simulink model "gm_Model"  (R2025a)
settings: Solver=FixedStepDiscrete  StartTime=0.0  StopTime=80000/fs_in  RelTol=1e-3
undefined symbols (not defined in the file or in its folder): a, b, b_fixp, beta_retanh, c, cos_omega, cos_omega_fixp, diag_count, exp_omega, exp_omega_fixp, fixp_chebacc_frac, fixp_chebacc_ws, fixp_dsp_ws, fixp_eig_frac, fixp_eig_ws, fs_in, group_size, hann_table_fixp, image_seed, image_seed_fixp, J_ROM, k, K_ROM, lap_diags, lap_main, lap_main_fi, lap_offsets, lap_offsets_fi, lap_rest, lap_rest_fi, laplacian_diags_main, laplacian_diags_offsets, laplacian_diags_rest, lut_norm_x, lut_norm_y, magnitude, n_ch, n_layer, n_px, n_px_fi, nf, norm_gain_floor, power_iters, power_norm_scaling_factor_fixp, tau, tau_fixp, theta, theta_fixp
libraries: simulink x59, hdlsllib x36, hdlstreaminglib x4, hdlmdlgenlib x1, matrix_library x1, dspvision x1
(part 4 of 8)

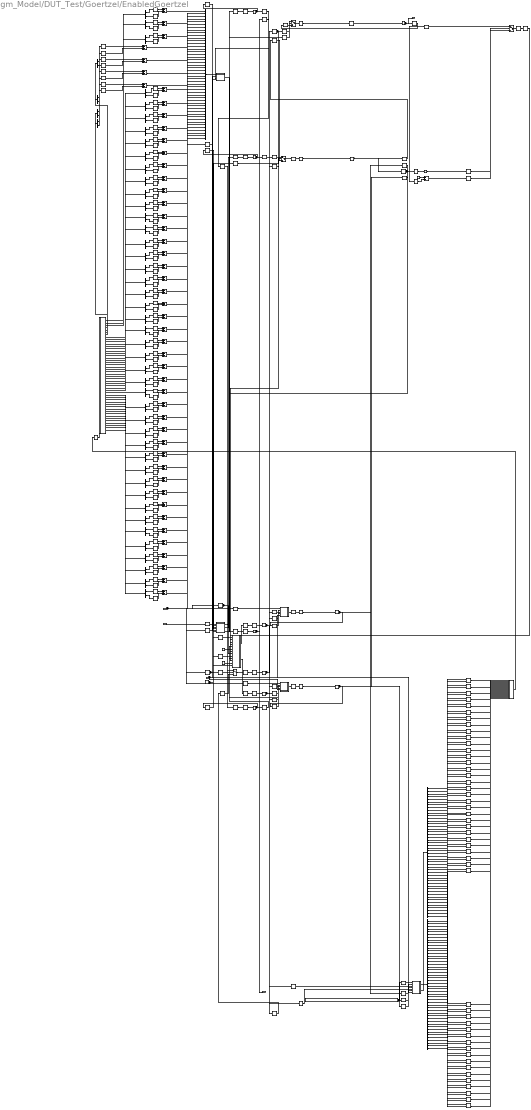
== system gm_Model/DUT_Test/Goertzel/EnabledGoertzel ==
  note: For Each
  note: For Each
  note: Symmetric Hann
  samples_in : Inport  OutDataTypeStr=fixdt(1, 12, 11)  PortDimensions=[1 48]  SampleTime=6.25e-05
  valid_in : Inport  Port=2  OutDataTypeStr=boolean  SampleTime=6.25e-05
  sch_ctr_199 : Inport  Port=3  OutDataTypeStr=uint8  SampleTime=3.125e-07
  Compare To Constant : simulink/Logic and Bit Operations/Compare To Constant  relop=<  const="fi(0,0,8,0,\"hex\",\"64\")"  OutDataTypeStr=boolean
  Constant : Constant  Value=[1.580322265625;1.6180419921875]  OutDataTypeStr=fixdt(1, 18, 13)  SampleTime=3.125e-07
  Constant1 : Constant  Value=0  OutDataTypeStr=fixdt(1, 18, 13)  SampleTime=3.125e-07
  Constant11 : Constant  Value=0  OutDataTypeStr=fixdt(1, 18, 13)  SampleTime=3.125e-07
  Constant12 : Constant  Value="complex(fi(\"numerictype\",numerictype(1,18,13),\"fimath\",fimath(\"RoundingMethod\", \"Nearest\",\"OverflowAction\", \"Saturate\",\"ProductMode\",\"FullPrecision\",\"SumMode\",\"FullPrecision\"),\"Value\",\"[0.7901611328125+0.6129150390625i;0.8089599609375+0.5877685546875i]\"))"  OutDataTypeStr=fixdt(1, 18, 13)  SampleTime=3.125e-07
  Constant2 : Constant  Value=199  OutDataTypeStr=uint8  SampleTime=3.125e-07
  Delay{,1..5,11..12,31,41} (10 alike) : RateTransition  InitialCondition=double(0)  OutPortSampleTimeOpt=Multiple of input port sample time  OutPortSampleTimeMultiple=200
  Delay1_absorbed : Delay  DelayLength=0
  Delay1_absorbed1 : Delay  DelayLength=0
  Delay1_absorbed2 : Delay  DelayLength=0
  Delay2_absorbed : Delay  DelayLength=0
  Delay2_enbsw : Switch  Criteria=u2 ~= 0  Threshold=double(0)  OutDataTypeStr=uint8  SampleTime=3.125e-07  SaturateOnIntegerOverflow=off  InputSameDT=off
  Delay3_absorbed : Delay  DelayLength=0
  Delay4_absorbed : Delay  DelayLength=0
  Delay4_enbsw : Switch  Criteria=u2 ~= 0  Threshold=double(0)  OutDataTypeStr=boolean  SampleTime=3.125e-07  SaturateOnIntegerOverflow=off  InputSameDT=off
  Delay_absorbed{,1..3} (4 alike) : Delay  DelayLength=0
  Delay_enbsw : Switch  Criteria=u2 ~= 0  Threshold=double(0)  OutDataTypeStr=boolean  SampleTime=3.125e-07  SaturateOnIntegerOverflow=off  InputSameDT=off
  HDL Counter : RateTransition  InitialCondition=double(0)  OutPortSampleTimeOpt=Multiple of input port sample time  OutPortSampleTimeMultiple=200
  HDL Counter_absorbed : Delay  DelayLength=0
  Hann : Subsystem
  Selector_1 : Selector  InputPortWidth=2  IndexOptions=Index vector (dialog)  Indices=double(1)  OutputSizes=1
  Selector_11 : Selector  InputPortWidth=2  IndexOptions=Index vector (dialog)  Indices=double(1)  OutputSizes=1
  Selector_2 : Selector  InputPortWidth=2  IndexOptions=Index vector (dialog)  Indices=double(2)  OutputSizes=1
  Selector_21 : Selector  InputPortWidth=2  IndexOptions=Index vector (dialog)  Indices=double(2)  OutputSizes=1
  Sum : Sum  Inputs=+-  OutDataTypeStr=uint8  AccumDataTypeStr=uint8  SampleTime=3.125e-07
  Sum of Elements_stage{2,21..29,210..247} (48 alike) : Sum  OutDataTypeStr=fixdt(1, 18, 13)  AccumDataTypeStr=fixdt(1, 18, 13)  SampleTime=3.125e-07
  Switch : Switch  Criteria=u2 ~= 0  Threshold="fi(0,0,1,0,\"hex\",\"0\")"  OutDataTypeStr=uint8  SampleTime=3.125e-07  SaturateOnIntegerOverflow=off  InputSameDT=off
  concatenate{,1..47} (48 alike) : Concatenate  ConcatenateDimension=2
  concatenate48 : Concatenate  NumInputs=48  Mode=Multidimensional array  ConcatenateDimension=2
  crp_out_delay{,1..10} (11 alike) : Delay  DelayLength=double(1)  InitialCondition=0
  crp_temp_streamed : Subsystem
  crp_temp_streamed1 : Subsystem
  crp_temp_streamed2 : Subsystem
  in0_repeat{,1..5} (6 alike) : RateTransition  Integrity=off  Deterministic=off  OutPortSampleTimeOpt=Multiple of input port sample time  OutPortSampleTimeMultiple=1/200
  in1_repeat{,1..5} (6 alike) : RateTransition  Integrity=off  Deterministic=off  OutPortSampleTimeOpt=Multiple of input port sample time  OutPortSampleTimeMultiple=1/200
  in2_repeat{,1..5} (6 alike) : RateTransition  Integrity=off  Deterministic=off  OutPortSampleTimeOpt=Multiple of input port sample time  OutPortSampleTimeMultiple=1/200
  in3_repeat{,1..5} (6 alike) : RateTransition  Integrity=off  Deterministic=off  OutPortSampleTimeOpt=Multiple of input port sample time  OutPortSampleTimeMultiple=1/200
  in4_repeat{,1..3} (4 alike) : RateTransition  Integrity=off  Deterministic=off  OutPortSampleTimeOpt=Multiple of input port sample time  OutPortSampleTimeMultiple=1/200
  in5_repeat : RateTransition  Integrity=off  Deterministic=off  OutPortSampleTimeOpt=Multiple of input port sample time  OutPortSampleTimeMultiple=1/200
  in5_repeat1 : RateTransition  Integrity=off  Deterministic=off  OutPortSampleTimeOpt=Multiple of input port sample time  OutPortSampleTimeMultiple=1/200
  in6_repeat : RateTransition  Integrity=off  Deterministic=off  OutPortSampleTimeOpt=Multiple of input port sample time  OutPortSampleTimeMultiple=1/200
  in7_repeat : RateTransition  Integrity=off  Deterministic=off  OutPortSampleTimeOpt=Multiple of input port sample time  OutPortSampleTimeMultiple=1/200
  in8_repeat : RateTransition  Integrity=off  Deterministic=off  OutPortSampleTimeOpt=Multiple of input port sample time  OutPortSampleTimeMultiple=1/200
  mux : Mux  Inputs=48
  rd_{0..40,42..96,111,121,210..211,410..411,511,531,611,621,710,810} (108 alike) : Delay  DelayLength=double(1)  InitialCondition=0
  rd_01 : Delay  DelayLength=double(1)  InitialCondition=0
  rd_02 : Delay  DelayLength=double(1)  InitialCondition=0
  rd_41 : Delay  DelayLength=double(2)  InitialCondition=0
  streaming_partition_streamed : Subsystem
  streaming_partition_streamed1 : Subsystem
  streaming_partition_streamed2 : Subsystem
  t : Demux  Outputs=48
  t1 : Demux  Outputs=48
  t{3..50} (48 alike) : Demux  Outputs=2
  t2 : Subsystem
  t51 : Reshape  OutputDimensionality=Customize  OutputDimensions=[2,48]
  valid_out : Outport  SampleTime=6.25e-05
  Out1 : Outport  Port=2  SampleTime=6.25e-05
  wires:
  streaming_partition_streamed/1(out0) -> crp_out_delay9/1
  rd_55/1 -> Sum of Elements_stage27/2
  t2/3(out2) -> t5/1
  t44/2 -> rd_89/1
  rd_7/1 -> Sum/2
  concatenate12/1 -> concatenate48/15
  crp_out_delay3/1 -> Delay3/1
  crp_out_delay10/1 -> Delay31/1
  streaming_partition_streamed1/1(out0) -> crp_out_delay10/1
  t22/1 -> rd_19/1
  t1/16 -> concatenate13/1
  crp_out_delay/1 -> Delay1/1
  rd_61/1 -> Switch/2
  t1/20 -> concatenate17/1
  t31/1 -> rd_28/1
  rd_16/1 -> Sum of Elements_stage216/1
  t/30 -> concatenate27/2
  crp_temp_streamed2/1(out0) -> crp_out_delay6/1
  Sum of Elements_stage228/1 -> mux/29
  rd_64/1 -> Sum of Elements_stage216/2
  rd_21/1 -> Delay4_enbsw/3
  Sum of Elements_stage240/1 -> mux/41
  crp_temp_streamed1/1(out0) -> crp_out_delay5/1
  rd_19/1 -> Sum of Elements_stage219/1
  crp_out_delay9/1 -> Delay12/1
  t8/1 -> rd_53/1
  t1/23 -> concatenate20/1
  rd_78/1 -> Sum of Elements_stage230/2
  rd_9/1 -> Hann/1(In1)
  Sum of Elements_stage238/1 -> mux/39
  rd_611/1 -> Sum of Elements_stage213/2
  rd_621/1 -> Sum of Elements_stage214/2
  concatenate34/1 -> concatenate48/37
  rd_63/1 -> Sum of Elements_stage215/2
  rd_96/1 -> Sum of Elements_stage29/1
  t2/1(out0) -> t3/1
  Sum of Elements_stage27/1 -> mux/8
  t42/1 -> rd_39/1
  t/28 -> concatenate25/2
  rd_10/1 -> Sum of Elements_stage210/1
  t/26 -> concatenate23/2
  t10/2 -> rd_55/1
  t2/33(out32) -> t35/1
  rd_44/1 -> Sum of Elements_stage244/1
  t19/1 -> rd_16/1
  rd_02/1 -> Sum of Elements_stage2/1
  concatenate45/1 -> concatenate48/48
  t33/1 -> rd_30/1
  in3_repeat4/1 -> crp_temp_streamed2/4(in3)
  t/22 -> concatenate19/2
  in4_repeat2/1 -> rd_4/1
  Delay5/1 -> Delay_absorbed3/1
  rd_13/1 -> Sum of Elements_stage213/1
  rd_14/1 -> Sum of Elements_stage214/1
  rd_52/1 -> Sum of Elements_stage24/2
  rd_15/1 -> Sum of Elements_stage215/1
  rd_68/1 -> Sum of Elements_stage220/2
  t1/27 -> concatenate24/1
  rd_810/1 -> Sum of Elements_stage28/1
  concatenate41/1 -> concatenate48/44
  t1/31 -> concatenate28/1
  rd_45/1 -> Sum of Elements_stage245/1
  in4_repeat/1 -> streaming_partition_streamed2/2(in1)
  rd_46/1 -> Sum of Elements_stage246/1
  rd_60/1 -> Sum of Elements_stage212/2
  rd_91/1 -> Sum of Elements_stage243/2
  t2/6(out5) -> t8/1
  t37/2 -> rd_82/1
  rd_82/1 -> Sum of Elements_stage234/2
  crp_temp_streamed/3(out2) -> crp_out_delay2/1
  rd_121/1 -> Sum of Elements_stage212/1
  t/34 -> concatenate31/2
  t28/1 -> rd_25/1
  Constant12/1 -> Selector_11/1, Selector_21/1
  rd_95/1 -> Sum of Elements_stage247/2
  t2/41(out40) -> t43/1
  rd_94/1 -> Sum of Elements_stage246/2
  concatenate15/1 -> concatenate48/18
  rd_25/1 -> Sum of Elements_stage225/1
  rd_58/1 -> Sum of Elements_stage210/2
  t1/12 -> concatenate9/1
  rd_59/1 -> Sum of Elements_stage211/2
  rd_36/1 -> Sum of Elements_stage236/1
  in1_repeat2/1 -> rd_5/1, rd_1/1
  t2/20(out19) -> t22/1
  t1/13 -> concatenate10/1
  rd_111/1 -> Sum of Elements_stage211/1
  t27/2 -> rd_72/1
  t2/18(out17) -> t20/1
  t25/2 -> rd_70/1
  Sum of Elements_stage220/1 -> mux/21
  t1/41 -> concatenate38/1
  t1/26 -> concatenate23/1
  in8_repeat/1 -> rd_41/1, rd_51/1, rd_7/1
  rd_57/1 -> Sum of Elements_stage29/2
  concatenate35/1 -> concatenate48/38
  mux/1 -> streaming_partition_streamed1/1(in0)
  Delay4_enbsw/1 -> crp_out_delay7/1
  t2/46(out45) -> t48/1
  rd_35/1 -> Sum of Elements_stage235/1
  t5/2 -> rd_50/1
  t2/38(out37) -> t40/1
  concatenate30/1 -> concatenate48/33
  t2/2(out1) -> t4/1
  t50/1 -> rd_47/1
  rd_92/1 -> Sum of Elements_stage244/2
  t2/23(out22) -> t25/1
  t1/37 -> concatenate34/1
  in1_repeat/1 -> rd_11/1, streaming_partition_streamed/8(in7)
  rd_23/1 -> Sum of Elements_stage223/1
  t24/2 -> rd_69/1
  t35/2 -> rd_80/1
  rd_41/1 -> Switch/1
  t2/12(out11) -> t14/1
  Delay4_absorbed/1 -> in2_repeat5/1, valid_out/1
  rd_511/1 -> Sum of Elements_stage23/2
  t1/47 -> concatenate44/1
  rd_62/1 -> Sum of Elements_stage26/1
  t1/36 -> concatenate33/1
  rd_210/1 -> Sum of Elements_stage22/1
  rd_56/1 -> Sum of Elements_stage28/2
  t21/1 -> rd_18/1
  t1/24 -> concatenate21/1
  t2/16(out15) -> t18/1
  rd_11/1 -> Delay4_enbsw/2
  sch_ctr_199/1 -> crp_temp_streamed2/5(enb_counter), crp_temp_streamed1/5(enb_counter), streaming_partition_streamed1/4(enb_counter), streaming_partition_streamed2/7(enb_counter), crp_temp_streamed/6(enb_counter), streaming_partition_streamed/13(enb_counter)
  t31/2 -> rd_76/1
  rd_4/1 -> Delay2_enbsw/1
  rd_710/1 -> Sum of Elements_stage27/1
  rd_01/1 -> Delay4_enbsw/1
  Sum of Elements_stage235/1 -> mux/36
  rd_37/1 -> Sum of Elements_stage237/1
  rd_17/1 -> Sum of Elements_stage217/1
  rd_54/1 -> Sum of Elements_stage26/2
  t1/35 -> concatenate32/1
  rd_43/1 -> Sum of Elements_stage243/1
  t47/2 -> rd_92/1
  crp_temp_streamed/2(out1) -> crp_out_delay1/1
  in2_repeat3/1 -> crp_temp_streamed/3(in2)
  t32/1 -> rd_29/1
  t/47 -> concatenate44/2
  Sum of Elements_stage222/1 -> mux/23
  streaming_partition_streamed2/1(out0) -> t/1
  Delay3_absorbed/1 -> Out1/1, in1_repeat5/1
  rd_531/1 -> Sum of Elements_stage25/2
  rd_1/1 -> Delay_enbsw/2
  rd_53/1 -> Sum of Elements_stage25/1
  t/11 -> concatenate8/2
  rd_89/1 -> Sum of Elements_stage241/2
  t6/1 -> rd_3/1
  t2/44(out43) -> t46/1
  t/15 -> concatenate12/2
  t3/2 -> rd_48/1
  rd_410/1 -> Sum of Elements_stage24/1
  rd_87/1 -> Sum of Elements_stage239/2
  t2/31(out30) -> t33/1
  t16/2 -> rd_611/1
  t2/24(out23) -> t26/1
  t1/45 -> concatenate42/1
  t23/2 -> rd_68/1
  rd_3/1 -> Sum of Elements_stage23/1
  Selector_11/1 -> streaming_partition_streamed2/4(in3)
  t2/42(out41) -> t44/1
  Sum of Elements_stage227/1 -> mux/28
  rd_411/1 -> Sum of Elements_stage241/1
  t38/1 -> rd_35/1
  rd_50/1 -> Sum of Elements_stage22/2
  t34/1 -> rd_31/1
  rd_38/1 -> Sum of Elements_stage238/1
  rd_0/1 -> Delay_enbsw/1
  in3_repeat/1 -> streaming_partition_streamed2/6(in5)
  t34/2 -> rd_79/1
  t2/9(out8) -> t11/1
  t/5 -> concatenate2/2
  rd_49/1 -> Sum of Elements_stage21/2
  rd_12/1 -> Sum of Elements_stage21/1
  Delay2_absorbed/1 -> in3_repeat2/1, in8_repeat/1
  rd_48/1 -> Sum of Elements_stage2/2
  concatenate40/1 -> concatenate48/43
  rd_86/1 -> Sum of Elements_stage238/2
  rd_47/1 -> Sum of Elements_stage247/1
  Delay4/1 -> Delay_absorbed2/1
  Delay_absorbed1/1 -> in2_repeat1/1, in2_repeat4/1, in0_repeat3/1, in2_repeat2/1
  Sum of Elements_stage210/1 -> mux/11
  rd_93/1 -> Sum of Elements_stage245/2
  in1_repeat4/1 -> crp_temp_streamed2/2(in1)
  rd_74/1 -> Sum of Elements_stage226/2
  in0_repeat3/1 -> rd_01/1, streaming_partition_streamed/7(in6)
  concatenate29/1 -> concatenate48/32
  rd_40/1 -> Sum of Elements_stage240/1
  t25/1 -> rd_22/1
  t/46 -> concatenate43/2
  streaming_partition_streamed2/2(out1) -> t1/1
  rd_90/1 -> Sum of Elements_stage242/2
  rd_42/1 -> Sum of Elements_stage242/1
  rd_88/1 -> Sum of Elements_stage240/2
  Constant2/1 -> Sum/1
  concatenate6/1 -> concatenate48/9
  t8/2 -> rd_531/1
  t2/39(out38) -> t41/1
  rd_39/1 -> Sum of Elements_stage239/1
  rd_85/1 -> Sum of Elements_stage237/2
  rd_84/1 -> Sum of Elements_stage236/2
  t/41 -> concatenate38/2
  t5/1 -> rd_210/1
  rd_83/1 -> Sum of Elements_stage235/2
  t39/2 -> rd_84/1
  t2/8(out7) -> t10/1
  t17/1 -> rd_14/1
  concatenate48/1 -> t51/1
  concatenate17/1 -> concatenate48/20
  t46/1 -> rd_43/1
  rd_34/1 -> Sum of Elements_stage234/1
  t1/4 -> concatenate1/1
  t51/1 -> t2/1(in0)
  rd_81/1 -> Sum of Elements_stage233/2
  t1/17 -> concatenate14/1
  Sum of Elements_stage219/1 -> mux/20
  t48/2 -> rd_93/1
  rd_33/1 -> Sum of Elements_stage233/1
  rd_80/1 -> Sum of Elements_stage232/2
  Sum of Elements_stage236/1 -> mux/37
  t/36 -> concatenate33/2
  rd_32/1 -> Sum of Elements_stage232/1
  t39/1 -> rd_36/1
  rd_79/1 -> Sum of Elements_stage231/2
  t2/21(out20) -> t23/1
  t1/21 -> concatenate18/1
  t22/2 -> rd_67/1
  rd_31/1 -> Sum of Elements_stage231/1
  t35/1 -> rd_32/1
  rd_30/1 -> Sum of Elements_stage230/1
  Sum of Elements_stage214/1 -> mux/15
  rd_77/1 -> Sum of Elements_stage229/2
  concatenate23/1 -> concatenate48/26
  rd_70/1 -> Sum of Elements_stage222/2
  t12/1 -> rd_96/1
  rd_29/1 -> Sum of Elements_stage229/1
  t2/22(out21) -> t24/1
  t1/29 -> concatenate26/1
  t21/2 -> rd_66/1
  t2/48(out47) -> t50/1
  t/31 -> concatenate28/2
  rd_2/1 -> Delay_enbsw/3
  t/9 -> concatenate6/2
  rd_76/1 -> Sum of Elements_stage228/2
  rd_28/1 -> Sum of Elements_stage228/1
  t47/1 -> rd_44/1
  concatenate39/1 -> concatenate48/42
  rd_75/1 -> Sum of Elements_stage227/2
  rd_27/1 -> Sum of Elements_stage227/1
  Delay_absorbed3/1 -> in5_repeat/1, in6_repeat/1, in1_repeat4/1
  rd_26/1 -> Sum of Elements_stage226/1
  t1/22 -> concatenate19/1
  rd_73/1 -> Sum of Elements_stage225/2
  t1/28 -> concatenate25/1
  t/25 -> concatenate22/2
  rd_72/1 -> Sum of Elements_stage224/2
  concatenate44/1 -> concatenate48/47
  t1/2 -> concatenate46/1
  rd_24/1 -> Sum of Elements_stage224/1
  rd_71/1 -> Sum of Elements_stage223/2
  t/4 -> concatenate1/2
  rd_22/1 -> Sum of Elements_stage222/1
  rd_69/1 -> Sum of Elements_stage221/2
  crp_out_delay8/1 -> Delay11/1
  rd_211/1 -> Sum of Elements_stage221/1
  t26/1 -> rd_23/1
  t/38 -> concatenate35/2
  rd_20/1 -> Sum of Elements_stage220/1
  in5_repeat1/1 -> streaming_partition_streamed/2(in1)
  t2/37(out36) -> t39/1
  t6/2 -> rd_511/1
  rd_67/1 -> Sum of Elements_stage219/2
  concatenate16/1 -> concatenate48/19
  rd_66/1 -> Sum of Elements_stage218/2
  in2_repeat4/1 -> rd_2/1
  rd_18/1 -> Sum of Elements_stage218/1
  t/7 -> concatenate4/2
  Switch/1 -> rd_9/1
  t38/2 -> rd_83/1
  rd_65/1 -> Sum of Elements_stage217/2
  concatenate7/1 -> concatenate48/10
  t15/1 -> rd_121/1
  t20/2 -> rd_65/1
  t2/27(out26) -> t29/1
  concatenate26/1 -> concatenate48/29
  t50/2 -> rd_95/1
  t4/1 -> rd_12/1
  concatenate20/1 -> concatenate48/23
  t49/2 -> rd_94/1
  t49/1 -> rd_46/1
  t15/2 -> rd_60/1
  t2/32(out31) -> t34/1
  t48/1 -> rd_45/1
  concatenate13/1 -> concatenate48/16
  t13/2 -> rd_58/1
  t2/30(out29) -> t32/1
  Delay_absorbed2/1 -> in1_repeat3/1, in7_repeat/1, in3_repeat/1
  t46/2 -> rd_91/1
  t45/2 -> rd_90/1
  concatenate10/1 -> concatenate48/13
  t/42 -> concatenate39/2
  t45/1 -> rd_42/1
  t44/1 -> rd_411/1
  t2/4(out3) -> t6/1
  t43/2 -> rd_88/1
  Sum of Elements_stage24/1 -> mux/5
  t43/1 -> rd_40/1
  t1/43 -> concatenate40/1
  Selector_21/1 -> streaming_partition_streamed2/1(in0)
  t42/2 -> rd_87/1
  t41/2 -> rd_86/1
  t41/1 -> rd_38/1
  t14/2 -> rd_59/1
  t2/29(out28) -> t31/1
  t40/2 -> rd_85/1
  concatenate32/1 -> concatenate48/35
  t/24 -> concatenate21/2
  t40/1 -> rd_37/1
  Sum of Elements_stage28/1 -> mux/9
  Compare To Constant/1 -> rd_61/1
  crp_out_delay2/1 -> Delay/1
  Hann/1(Out1) -> streaming_partition_streamed/4(in3)
  t37/1 -> rd_34/1
  t2/11(out10) -> t13/1
  t36/2 -> rd_81/1
  t36/1 -> rd_33/1
  t/20 -> concatenate17/2
  Delay1_absorbed/1 -> in2_repeat3/1, in4_repeat1/1
  Delay3/1 -> Delay_absorbed1/1
  t2/28(out27) -> t30/1
  t19/2 -> rd_64/1
  t20/1 -> rd_17/1
  t2/10(out9) -> t12/1
  t33/2 -> rd_78/1
  t2/35(out34) -> t37/1
  t12/2 -> rd_57/1
  Sum of Elements_stage242/1 -> mux/43
  Sum of Elements_stage239/1 -> mux/40
  Sum of Elements_stage213/1 -> mux/14
  t2/15(out14) -> t17/1
  t32/2 -> rd_77/1
  Sum of Elements_stage226/1 -> mux/27
  t2/13(out12) -> t15/1
  t30/2 -> rd_75/1
  t/10 -> concatenate7/2
  t30/1 -> rd_27/1
  Sum of Elements_stage21/1 -> mux/2
  t2/14(out13) -> t16/1
  t29/2 -> rd_74/1
  t/8 -> concatenate5/2
  t29/1 -> rd_26/1
  t2/19(out18) -> t21/1
  t1/5 -> concatenate2/1
  t28/2 -> rd_73/1
  in3_repeat3/1 -> crp_temp_streamed1/4(in3)
  t/37 -> concatenate34/2
  crp_temp_streamed/1(out0) -> crp_out_delay/1
  t27/1 -> rd_24/1
  t1/8 -> concatenate5/1
  t/43 -> concatenate40/2
  t2/17(out16) -> t19/1
  t26/2 -> rd_71/1
  concatenate21/1 -> concatenate48/24
  t9/1 -> rd_62/1
  Sum of Elements_stage2/1 -> mux/1
  t/17 -> concatenate14/2
  t24/1 -> rd_211/1
  t1/32 -> concatenate29/1
  t1/46 -> concatenate43/1
  t23/1 -> rd_20/1
  t1/40 -> concatenate37/1
  t18/2 -> rd_63/1
  concatenate/1 -> concatenate48/3
  t2/25(out24) -> t27/1
  t18/1 -> rd_15/1
  t1/48 -> concatenate45/1
  t2/26(out25) -> t28/1
  t17/2 -> rd_621/1
  t16/1 -> rd_13/1
  crp_out_delay4/1 -> Delay2/1
  Sum of Elements_stage233/1 -> mux/34
  t14/1 -> rd_111/1
  concatenate14/1 -> concatenate48/17
  t13/1 -> rd_10/1
  t2/36(out35) -> t38/1
  concatenate1/1 -> concatenate48/4
  t11/2 -> rd_56/1
  t11/1 -> rd_810/1
  Sum of Elements_stage245/1 -> mux/46
  t10/1 -> rd_710/1
  t/19 -> concatenate16/2
  t2/34(out33) -> t36/1
  t9/2 -> rd_54/1
  in2_repeat5/1 -> rd_21/1
  t2/40(out39) -> t42/1
  t7/2 -> rd_52/1
  t7/1 -> rd_410/1
  t/2 -> concatenate46/2
  t2/43(out42) -> t45/1
  t4/2 -> rd_49/1
  concatenate19/1 -> concatenate48/22
  concatenate8/1 -> concatenate48/11
  t3/1 -> rd_02/1
  Sum of Elements_stage247/1 -> mux/48
  in1_repeat5/1 -> streaming_partition_streamed1/3(in2)
  Sum of Elements_stage22/1 -> mux/3
  concatenate3/1 -> concatenate48/6
  Sum of Elements_stage246/1 -> mux/47
  t1/44 -> concatenate41/1
  Sum of Elements_stage244/1 -> mux/45
  Delay_enbsw/1 -> crp_out_delay3/1
  Sum of Elements_stage243/1 -> mux/44
  concatenate28/1 -> concatenate48/31
  Sum of Elements_stage241/1 -> mux/42
  t1/7 -> concatenate4/1
  in2_repeat1/1 -> crp_temp_streamed1/3(in2)
  Sum of Elements_stage237/1 -> mux/38
  Sum of Elements_stage234/1 -> mux/35
  concatenate25/1 -> concatenate48/28
  Sum of Elements_stage29/1 -> mux/10
  concatenate2/1 -> concatenate48/5
  Sum of Elements_stage232/1 -> mux/33
  Sum of Elements_stage23/1 -> mux/4
  Sum of Elements_stage231/1 -> mux/32
  Sum of Elements_stage230/1 -> mux/31
  Delay1_absorbed1/1 -> in2_repeat/1, in3_repeat3/1, in3_repeat5/1
  Sum of Elements_stage229/1 -> mux/30
  t1/1 -> concatenate47/1
  Sum of Elements_stage225/1 -> mux/26
  t1/9 -> concatenate6/1
  Sum of Elements_stage224/1 -> mux/25
  t/39 -> concatenate36/2
  Sum of Elements_stage223/1 -> mux/24
  t1/33 -> concatenate30/1
  Sum of Elements_stage221/1 -> mux/22
  t1/25 -> concatenate22/1
  Sum of Elements_stage218/1 -> mux/19
  Sum of Elements_stage217/1 -> mux/18
  Sum of Elements_stage216/1 -> mux/17
  Constant11/1 -> streaming_partition_streamed/6(in5)
  Sum of Elements_stage215/1 -> mux/16
  Sum of Elements_stage212/1 -> mux/13
  samples_in/1 -> in0_repeat4/1
  Sum of Elements_stage211/1 -> mux/12
  concatenate31/1 -> concatenate48/34
  t/33 -> concatenate30/2
  concatenate24/1 -> concatenate48/27
  HDL Counter_absorbed/1 -> in3_repeat1/1, in4_repeat2/1
  t2/47(out46) -> t49/1
  t2/45(out44) -> t47/1
  t/13 -> concatenate10/2
  concatenate46/1 -> concatenate48/2
  concatenate33/1 -> concatenate48/36
  concatenate22/1 -> concatenate48/25
  crp_out_delay7/1 -> Delay41/1
  concatenate47/1 -> concatenate48/1
  Constant/1 -> Selector_2/1, Selector_1/1
  t1/42 -> concatenate39/1
  t1/39 -> concatenate36/1
  t1/38 -> concatenate35/1
  t1/34 -> concatenate31/1
  concatenate18/1 -> concatenate48/21
  in4_repeat3/1 -> crp_temp_streamed/5(in4)
  t1/30 -> concatenate27/1
  concatenate5/1 -> concatenate48/8
  concatenate42/1 -> concatenate48/45
  t1/19 -> concatenate16/1
  t1/18 -> concatenate15/1
  concatenate27/1 -> concatenate48/30
  Delay12/1 -> Delay1_absorbed2/1
  Delay/1 -> Delay_absorbed/1
  t1/15 -> concatenate12/1
  t1/14 -> concatenate11/1
  in0_repeat/1 -> streaming_partition_streamed1/2(in1)
  t1/11 -> concatenate8/1
  t/27 -> concatenate24/2
  t1/10 -> concatenate7/1
  t1/6 -> concatenate3/1
  t1/3 -> concatenate/1
  t/48 -> concatenate45/2
  t/45 -> concatenate42/2
  in4_repeat1/1 -> streaming_partition_streamed/5(in4)
  t/44 -> concatenate41/2
  t/40 -> concatenate37/2
  in1_repeat1/1 -> crp_temp_streamed/2(in1)
  in0_repeat4/1 -> crp_temp_streamed/1(in0)
  t/35 -> concatenate32/2
  t/32 -> concatenate29/2
  t/29 -> concatenate26/2
  t/23 -> concatenate20/2
  t/21 -> concatenate18/2
  t/18 -> concatenate15/2
  t/16 -> concatenate13/2
  rd_6/1 -> Delay2_enbsw/3
  t/14 -> concatenate11/2
  t/12 -> concatenate9/2
  t/6 -> concatenate3/2
  t/3 -> concatenate/2
  t/1 -> concatenate47/2
  concatenate43/1 -> concatenate48/46
  concatenate38/1 -> concatenate48/41
  concatenate37/1 -> concatenate48/40
  Delay2/1 -> Delay2_absorbed/1
  Delay31/1 -> Delay3_absorbed/1
  concatenate36/1 -> concatenate48/39
  concatenate11/1 -> concatenate48/14
  concatenate9/1 -> concatenate48/12
  concatenate4/1 -> concatenate48/7
  Delay1/1 -> Delay1_absorbed/1
  streaming_partition_streamed/2(out1) -> crp_out_delay8/1
  rd_51/1 -> Compare To Constant/1
  rd_8/1 -> Switch/3
  Sum/1 -> rd_8/1
  Selector_1/1 -> streaming_partition_streamed/9(in8)
  Selector_2/1 -> streaming_partition_streamed/1(in0)
  Constant1/1 -> streaming_partition_streamed/12(in11)
  Delay2_enbsw/1 -> crp_out_delay4/1
  in5_repeat/1 -> streaming_partition_streamed2/3(in2)
  Delay41/1 -> Delay4_absorbed/1
  Delay11/1 -> Delay1_absorbed1/1
  crp_out_delay6/1 -> Delay5/1
  in2_repeat2/1 -> crp_temp_streamed2/3(in2)
  in3_repeat1/1 -> crp_temp_streamed/4(in3)
  in1_repeat3/1 -> crp_temp_streamed1/2(in1)
  crp_out_delay5/1 -> Delay4/1
  crp_out_delay1/1 -> HDL Counter/1
  HDL Counter/1 -> HDL Counter_absorbed/1
  Delay_absorbed/1 -> in4_repeat3/1, in0_repeat5/1
  Delay1_absorbed2/1 -> in4_repeat/1, in3_repeat4/1, in5_repeat1/1
  valid_in/1 -> in0_repeat1/1, in0_repeat2/1, in1_repeat/1, in0_repeat/1, in1_repeat1/1, in1_repeat2/1
  in0_repeat1/1 -> crp_temp_streamed1/1(in0)
  Sum of Elements_stage26/1 -> mux/7
  Sum of Elements_stage25/1 -> mux/6
  in0_repeat2/1 -> crp_temp_streamed2/1(in0)
  rd_5/1 -> Delay2_enbsw/2
  in2_repeat/1 -> streaming_partition_streamed2/5(in4)
  in3_repeat5/1 -> streaming_partition_streamed/10(in9)
  in0_repeat5/1 -> rd_0/1
  in6_repeat/1 -> streaming_partition_streamed/3(in2)
  in3_repeat2/1 -> rd_6/1
  in7_repeat/1 -> streaming_partition_streamed/11(in10)
  t2/5(out4) -> t7/1
  t2/7(out6) -> t9/1

== system gm_Model/DUT_ref/Backprojection/For Each Subsystem ==
  In1 : Inport
  Complex to Real-Imag : ComplexToRealImag  Output=Real
  Constant : Constant  Value=b
  Constant1 : Constant  Value=tau
  For Each : ForEach  DisableCoverage=on  IterateSubsysMaskParameter=on,on  SubsysMaskParameterIterationDimension=2,2
  Hermitian : Math  Operator=hermitian
  Matrix Multiply : Product  Multiplication=Matrix(*)
  Matrix Multiply1 : Product  Multiplication=Matrix(*)
  Sum : Sum  Inputs=-+|
  Out1 : Outport  ConcatenationDimension=1
  wires:
  Sum/1 -> Out1/1
  Complex to Real-Imag/1 -> Sum/2
  Constant1/1 -> Sum/1
  Matrix Multiply1/1 -> Complex to Real-Imag/1
  Matrix Multiply/1 -> Matrix Multiply1/1
  In1/1 -> Matrix Multiply/2
  Constant/1 -> Hermitian/1, Matrix Multiply1/2
  Hermitian/1 -> Matrix Multiply/1

== system gm_Model/DUT_ref/CrossCor/Correlation ==
  In1 : Inport
  Math Function : Math  Operator=conj
  Math Function1 : Math  Operator=transpose
  Math Function2 : Math  Operator=transpose
  MatrixMultiply : Product  Multiplication=Matrix(*)
  in : Outport
  wires:
  Math Function1/1 -> Math Function/1, Math Function2/1
  Math Function2/1 -> MatrixMultiply/2
  Math Function/1 -> MatrixMultiply/1
  In1/1 -> Math Function1/1
  MatrixMultiply/1 -> in/1

== system gm_Model/DUT_ref/CrossCor/Grouping ==
  note: Sum 9 frames and reduce data rate
  en : Inport
  in : Inport  Port=2
  Add : Sum
  DataValidDownsampler : Subsystem  mask{rate_factor=group_size}
  Delay : Delay  DelayLength=1
  Delay1 : Delay  DelayLength=1
  HDL Counter : hdlsllib/Sources/HDL Counter  CountType=Count limited  CountInit=0  CountStep=1  CountMax=group_size-1  CountFromType=Initial value  CountFrom=0  CountResetPort=off  CountLoadPort=off  CountEnbPort=on  CountDirPort=off  CountHitOutputPort=on  CountDataType=Unsigned  CountWordLen=ceil(log2(group_size))  CountFracLen=0  CountSampTime=-1
  Real-Imag to Complex : RealImagToComplex
  Real-Imag to Complex1 : RealImagToComplex
  Switch : Switch  Criteria=u2 ~= 0  SaturateOnIntegerOverflow=off  InputSameDT=off
  Switch1 : Switch  Criteria=u2 ~= 0  SaturateOnIntegerOverflow=off  InputSameDT=off
  Terminator : Terminator
  Zero : Constant  Value=0  OutDataTypeStr=Inherit: Inherit via back propagation  SampleTime=-1
  Zero1 : Constant  Value=0  OutDataTypeStr=Inherit: Inherit via back propagation  SampleTime=-1
  valid : Outport
  out : Outport  Port=2
  wires:
  DataValidDownsampler/1(ValidSlow) -> valid/1
  DataValidDownsampler/2(DataSlow) -> out/1
  HDL Counter/1 -> Terminator/1
  Real-Imag to Complex1/1 -> Switch1/3
  Zero1/1 -> Real-Imag to Complex1/1, Real-Imag to Complex1/2
  in/1 -> Switch1/1
  Switch1/1 -> Add/1
  en/1 -> HDL Counter/1, Switch1/2
  Real-Imag to Complex/1 -> Switch/1
  Switch/1 -> Add/2
  Delay/1 -> DataValidDownsampler/2(DataFast), Switch/3
  Add/1 -> Delay/1
  Delay1/1 -> Switch/2, DataValidDownsampler/1(ValidFast)
  Zero/1 -> Real-Imag to Complex/1, Real-Imag to Complex/2
  HDL Counter/2 -> Delay1/1

== system gm_Model/DUT_ref/CrossCor/NormalizationEigen ==
  In1 : Inport
      settings: SignalType=complex
  Constant : Constant  SampleTime=-1
  PowerIteration : Subsystem
  Product : Product
  Reciprocal : Product  Inputs=/
  Switch : Switch  Criteria=u2 > Threshold  SaturateOnIntegerOverflow=off  InputSameDT=off
  Out1 : Outport
  wires:
  PowerIteration/2(MaxEigenvalue) -> Switch/1, Switch/2
  Constant/1 -> Switch/3
  Switch/1 -> Reciprocal/1
  PowerIteration/1(MatOut) -> Product/1
  Reciprocal/1 -> Product/2
  Product/1 -> Out1/1
  In1/1 -> PowerIteration/1(MatIn)

== system gm_Model/DUT_ref/CrossCor/NormalizationPower ==
  out : Inport
      settings: SignalType=complex
  Complex to Real-Imag : ComplexToRealImag  Output=Real
  Delay1 : Delay  DelayLength=1
  Extract Diagonal : matrix_library/Extract Diagonal
      settings: LibrarySourceBlock=|
      | simulink/Matrix
      | Operations/Extract Diagonal
  Gain : Gain  Gain=1/sqrt(2)
  Product : Product
  Reciprocal : Product  Inputs=/
  Sum of Elements : Sum  Inputs=+
  data_out : Outport
  wires:
  Delay1/1 -> data_out/1
  Complex to Real-Imag/1 -> Sum of Elements/1
  Extract Diagonal/1 -> Complex to Real-Imag/1
  Sum of Elements/1 -> Gain/1
  Gain/1 -> Reciprocal/1
  out/1 -> Extract Diagonal/1, Product/1
  Reciprocal/1 -> Product/2
  Product/1 -> Delay1/1

== system gm_Model/DUT_ref/Deblurring/Chebyshev ==
  note: In to output delay (in slow IO speed): 1
  Image_in : Inport
  AccumulatorCounter : Subsystem
  Constant1 : Constant  Value=theta  SampleTime=-1
  Delay2 : Delay
  Gain1 : Gain  Gain=2
  Index Vector : MultiPortSwitch  DataPortOrder=Zero-based contiguous  DiagnosticForDefault=None  zeroidx=on  SaturateOnIntegerOverflow=off  InputSameDT=off
  LaplacianMultiply : Subsystem
  Rate Transition : RateTransition  Integrity=off  OutPortSampleTimeOpt=Multiple of input port sample time  OutPortSampleTimeMultiple=1/(k+1)
  Rate Transition2 : RateTransition  OutPortSampleTimeOpt=Multiple of input port sample time  OutPortSampleTimeMultiple=k+1
  Selector1 : Selector  IndexMode=Zero-based  InputPortWidth=k+1  IndexOptions=Index vector (port)  Indices=[1 3]  OutputSizes=1
  Sum1 : Sum  Inputs=|+-
  Out1 : Outport
  wires:
  [cheb_iter] -> Selector1/2
  AccumulatorCounter/1(counter) -> [cheb_iter]
  Constant1/1 -> Selector1/1
  Rate Transition2/1 -> Out1/1
  AccumulatorCounter/2(accum) -> Rate Transition2/1
  Selector1/1 -> AccumulatorCounter/1(a)
  [cheb_iter] -> Index Vector/1
  Image_in/1 -> Rate Transition/1
  Index Vector/1 -> AccumulatorCounter/2(b), Delay2/1, LaplacianMultiply/1(Image_in)  "z_k"
  Sum1/1 -> Index Vector/4
  LaplacianMultiply/1(Image_out) -> Index Vector/3, Gain1/1
  Delay2/1 -> Sum1/2  "z_k-2"
  Gain1/1 -> Sum1/1
  Rate Transition/1 -> Index Vector/2

== system gm_Model/DUT_ref/Goertzel/DataValidDownsampler ==
  ValidFast : Inport
  DataFast : Inport  Port=2
  DataInSW : Switch  Criteria=u2 ~= 0  SaturateOnIntegerOverflow=off  InputSameDT=off
  DataMem : Delay  DelayLength=1
  DataRT : RateTransition  Deterministic=off  OutPortSampleTimeOpt=Multiple of input port sample time  OutPortSampleTimeMultiple=nf
  RisingEdgeDetector : Subsystem
  Terminator : Terminator
  ValidMem : Delay  DelayLength=1  ShowEnablePort=on
      settings: InputPortMap=u0,e6
  ValidRT : RateTransition  Deterministic=off  OutPortSampleTimeOpt=Multiple of input port sample time  OutPortSampleTimeMultiple=nf
  ValidResetCounter : hdlsllib/Sources/HDL Counter  CountType=Count limited  CountInit=0  CountStep=1  CountMax=nf-1  CountFromType=Initial value  CountFrom=0  CountResetPort=off  CountLoadPort=off  CountEnbPort=off  CountDirPort=off  CountHitOutputPort=on  CountDataType=Unsigned  CountWordLen=12  CountFracLen=0  CountSampTime=-1
  ValidResetDelay : Delay  DelayLength=1
  ValidSampleOR : Logic  Operator=OR  IconShape=distinctive  AllPortsSameDT=off  OutDataTypeStr=boolean
  ValidSlow : Outport
  DataSlow : Outport  Port=2
  wires:
  ValidResetCounter/1 -> Terminator/1
  DataFast/1 -> DataInSW/1
  DataRT/1 -> DataSlow/1
  ValidRT/1 -> ValidSlow/1
  ValidMem/1 -> ValidRT/1
  ValidResetDelay/1 -> ValidSampleOR/2
  ValidResetCounter/2 -> ValidResetDelay/1
  ValidFast/1 -> RisingEdgeDetector/1(In1)
  RisingEdgeDetector/1(Out1) -> ValidMem/1, ValidSampleOR/1, DataInSW/2
  DataInSW/1 -> DataMem/1
  DataMem/1 -> DataInSW/3, DataRT/1
  ValidSampleOR/1 -> ValidMem/2

== system gm_Model/DUT_ref/Goertzel/EnabledGoertzel ==
  In2 : Inport
  valid_in : EnablePort
  Delay : Delay  DelayLength=1
  Goertzel filter : Subsystem  TreatAsAtomicUnit=on
  HDL Counter : hdlsllib/Sources/HDL Counter  CountType=Count limited  CountInit=0  CountStep=1  CountMax=nf-1  CountFromType=Initial value  CountFrom=0  CountResetPort=off  CountLoadPort=off  CountEnbPort=off  CountDirPort=off  CountHitOutputPort=on  CountDataType=Unsigned  CountWordLen=8  CountFracLen=0  CountSampTime=1/fs_in
  Product : Product
  State Control : StateControl  StateControl=Synchronous
  Symmetric Hann : Subsystem
  valid_out : Outport
  Out1 : Outport  Port=2
  wires:
  Delay/1 -> valid_out/1, Goertzel filter/Reset
  Goertzel filter/1(Out1) -> Out1/1
  In2/1 -> Product/2
  Symmetric Hann/1(Out1) -> Product/1
  Product/1 -> Goertzel filter/1(u)
  HDL Counter/1 -> Symmetric Hann/1(u)
  HDL Counter/2 -> Delay/1

== system gm_Model/Unused blocks/BackprojOpt/For Each Subsystem ==
  cc : Inport
  b : Inport  Port=2
  Complex to Real-Imag : ComplexToRealImag  Output=Real
  Conjugate : Math  Operator=conj  SignedPower=on  RndMeth=Zero
  Constant : Constant  Value=K
  Constant1 : Constant  Value=J
  For Each : ForEach  DisableCoverage=on  IterateSubsysMaskParameter=on,on
  Product : Product  Inputs=3
  Selector : Selector  NumberOfDimensions=2  InputPortWidth=3  IndexOptions=Index vector (port),Index vector (port)  Indices=J,K  OutputSizes=1,1
  Selector1 : Selector  InputPortWidth=n_ch  IndexOptions=Index vector (port)  Indices=J  OutputSizes=1
  Selector2 : Selector  InputPortWidth=n_ch  IndexOptions=Index vector (port)  Indices=J  OutputSizes=1
  Out1 : Outport  ConcatenationDimension=1
  wires:
  Constant1/1 -> Selector1/2, Selector/2
  Constant/1 -> Selector2/2, Selector/3
  Complex to Real-Imag/1 -> Out1/1
  Product/1 -> Complex to Real-Imag/1
  Selector2/1 -> Product/3
  b/1 -> Selector2/1, Selector1/1
  Conjugate/1 -> Product/1
  Selector1/1 -> Conjugate/1
  Selector/1 -> Product/2
  cc/1 -> Selector/1

== system gm_Model/DUT_FixP/CrossCor/Grouping/DataValidDownsampler ==
  ValidFast : Inport
  DataFast : Inport  Port=2
  DataInSW : Switch  Criteria=u2 ~= 0  SaturateOnIntegerOverflow=off  InputSameDT=off
  DataMem : Delay  DelayLength=1
  DataRT : RateTransition  OutPortSampleTimeOpt=Multiple of input port sample time  OutPortSampleTimeMultiple=rate_factor
  RisingEdgeDetector : Subsystem
  Terminator : Terminator
  ValidMem : Delay  DelayLength=1  ShowEnablePort=on
      settings: InputPortMap=u0,e6
  ValidRT : RateTransition  OutPortSampleTimeOpt=Multiple of input port sample time  OutPortSampleTimeMultiple=rate_factor
  ValidResetCounter : hdlsllib/Sources/HDL Counter  CountType=Count limited  CountInit=0  CountStep=1  CountMax=rate_factor-1  CountFromType=Initial value  CountFrom=0  CountResetPort=off  CountLoadPort=off  CountEnbPort=off  CountDirPort=off  CountHitOutputPort=on  CountDataType=Unsigned  CountWordLen=ceil(log2(rate_factor))  CountFracLen=0  CountSampTime=-1
  ValidResetDelay : Delay  DelayLength=1
  ValidSampleOR : Logic  Operator=OR  IconShape=distinctive  AllPortsSameDT=off  OutDataTypeStr=boolean
  ValidSlow : Outport
  DataSlow : Outport  Port=2
  wires:
  ValidResetCounter/1 -> Terminator/1
  DataFast/1 -> DataInSW/1
  DataRT/1 -> DataSlow/1
  ValidRT/1 -> ValidSlow/1
  ValidMem/1 -> ValidRT/1
  ValidResetDelay/1 -> ValidSampleOR/2
  ValidResetCounter/2 -> ValidResetDelay/1
  ValidFast/1 -> RisingEdgeDetector/1(In1)
  RisingEdgeDetector/1(Out1) -> ValidMem/1, ValidSampleOR/1, DataInSW/2
  DataInSW/1 -> DataMem/1
  DataMem/1 -> DataInSW/3, DataRT/1
  ValidSampleOR/1 -> ValidMem/2

== system gm_Model/DUT_FixP/CrossCor/NormalizationEig/PowerIteration ==
  note: Norm of vector: sum(sq(abs(v)))
  MatIn : Inport
  Compare To Constant : simulink/Logic and Bit Operations/Compare To Constant  relop=<=  const=fi(1/2,0,fixp_eig_ws, fixp_eig_frac)  OutDataTypeStr=boolean
  Complex to Real-Imag : ComplexToRealImag  Output=Real
  Constant : Constant  Value=fi(1/2+2^-fixp_eig_frac,0,fixp_eig_ws, fixp_eig_frac)  SampleTime=-1
  Delay : Delay  DelayLength=1  InitialCondition=0
  Delay1 : Delay  DelayLength=1
  Delay2 : Delay  DelayLength=1  InitialCondition=0
  Delay3 : Delay  DelayLength=1
  Delay4 : Delay  DelayLength=1
  HDL Counter : hdlsllib/Sources/HDL Counter  CountType=Count limited  CountInit=0  CountStep=1  CountMax=power_iters-1  CountFromType=Initial value  CountFrom=0  CountResetPort=off  CountLoadPort=off  CountEnbPort=off  CountDirPort=off  CountHitOutputPort=off  CountDataType=Unsigned  CountWordLen=6  CountFracLen=0  CountSampTime=group_size*nf/(fs_in*power_iters)
  Hermitian : Math  Operator=hermitian
  Matrix Multiply : Product  Multiplication=Matrix(*)  OutDataTypeStr=Inherit: Same as first input
  Matrix Multiply1 : Product  Multiplication=Matrix(*)  OutDataTypeStr=Inherit: Same as first input
  Matrix Multiply2 : Product  Multiplication=Matrix(*)  OutDataTypeStr=Inherit: Same as first input
  Multiply : Product  Inputs=**  OutDataTypeStr=Inherit: Same as first input
  NormReciprocalLUT : Lookup_n-D  Commented=on  NumberOfTableDimensions=1  LookupTableObject=FSds  BreakpointsForDimension1=lut_norm_x  BreakpointsForDimension1FirstPoint=10  BreakpointsForDimension2FirstPoint=10  BreakpointsForDimension1Spacing=12  BreakpointsForDimension2Spacing=12  BreakpointsForDimension1DataTypeStr=Inherit: Inherit from 'Breakpoint data'  Table=lut_norm_y  TableDataTypeStr=Inherit: Inherit from 'Table data'  ExtrapMethod=Clip  DiagnosticForOutOfRangeInput=Error  RemoveProtectionInput=on  UseLastTableValue=on  OutDataTypeStr=Inherit: Inherit from 'Table data'  RndMeth=Simplest
  Product : Product  OutDataTypeStr=Inherit: Same as first input
  Rate Transition : RateTransition  InitialCondition=1
  Rate Transition1 : RateTransition  Integrity=off  OutPortSampleTimeOpt=Multiple of input port sample time  OutPortSampleTimeMultiple=1/power_iters
  Rate Transition2 : RateTransition  InitialCondition=1
  Real-Imag to Complex : RealImagToComplex  Input=Real
  Reciprocal : Product  Inputs=/  OutDataTypeStr=fixdt(0,24,23)
  SeedEigenVec : Constant  Value=fi(ones(1,n_ch)'./sqrt(n_ch),1,fixp_dsp_ws,fixp_eig_frac)  VectorParams1D=off  OutDataTypeStr=Inherit: Inherit via back propagation  SampleTime=-1
  Square : Math  Operator=magnitude^2  OutDataTypeStr=fixdt(0,fixp_eig_ws,fixp_eig_frac)
  Sum of Elements : Sum  Inputs=+  AccumDataTypeStr=fixdt(0,fixp_eig_ws,fixp_eig_frac)  SaturateOnIntegerOverflow=on
  Switch : Switch  Criteria=u2 > Threshold  SaturateOnIntegerOverflow=off  InputSameDT=off
  Switch1 : Switch  Criteria=u2 ~= 0  SaturateOnIntegerOverflow=off  InputSameDT=off
  MatOut : Outport
  MaxEigenvalue : Outport  Port=2
  wires:
  Reciprocal/1 -> Multiply/2
  Delay4/1 -> MatOut/1
  Delay3/1 -> MaxEigenvalue/1
  Complex to Real-Imag/1 -> Product/2
  Rate Transition2/1 -> Product/1  "Norm"
  Square/1 -> Sum of Elements/1
  Switch1/1 -> NormReciprocalLUT/1, Reciprocal/1
  Delay2/1 -> Rate Transition2/1
  Product/1 -> Delay3/1
  Compare To Constant/1 -> Switch1/2
  Constant/1 -> Switch1/1
  Sum of Elements/1 -> Delay2/1, Compare To Constant/1, Switch1/3
  Matrix Multiply1/1 -> Matrix Multiply2/1
  Hermitian/1 -> Matrix Multiply1/1
  Real-Imag to Complex/1 -> Switch/3
  SeedEigenVec/1 -> Real-Imag to Complex/1
  Delay1/1 -> Delay4/1, Matrix Multiply1/2
  Matrix Multiply2/1 -> Complex to Real-Imag/1
  Multiply/1 -> Delay/1
  MatIn/1 -> Rate Transition1/1, Delay1/1
  Rate Transition1/1 -> Matrix Multiply/1
  Matrix Multiply/1 -> Multiply/1, Square/1
  HDL Counter/1 -> Switch/2
  Switch/1 -> Matrix Multiply/2
  Rate Transition/1 -> Hermitian/1, Matrix Multiply2/2
  Delay/1 -> Rate Transition/1, Switch/1

== system gm_Model/DUT_FixP/Deblurring/Chebyshev/AccumulatorCounter ==
  a : Inport
  b : Inport  Port=2
  AccTypeCastBack : DataTypeConversion  SaturateOnIntegerOverflow=off  RndMeth=Floor
  Delay : Delay  DelayLength=1
  Delay1 : Delay  DelayLength=1
  HDL Counter : hdlsllib/Sources/HDL Counter  CountType=Count limited  CountInit=0  CountStep=1  CountMax=k  CountFromType=Initial value  CountFrom=0  CountResetPort=off  CountLoadPort=off  CountEnbPort=off  CountDirPort=off  CountHitOutputPort=on  CountDataType=Unsigned  CountWordLen=ceil(log2(k+1))  CountFracLen=0  CountSampTime=-1
  Multiply-Add : hdlsllib/HDL Operations/Multiply-Add  Function=c+(a.*b)  datatype=fixdt(1,fixp_chebacc_ws,fixp_chebacc_frac)  DoSatur=off  FMA=off
  Switch : Switch  Criteria=u2 ~= 0  SaturateOnIntegerOverflow=off  InputSameDT=off
  Zero : Constant  Value=0  OutDataTypeStr=Inherit: Inherit via back propagation  SampleTime=-1
  counter : Outport
  accum : Outport  Port=2
  wires:
  AccTypeCastBack/1 -> accum/1
  b/1 -> Multiply-Add/2
  Switch/1 -> Multiply-Add/3
  Delay/1 -> AccTypeCastBack/1, Switch/3
  Multiply-Add/1 -> Delay/1
  Delay1/1 -> Switch/2
  Zero/1 -> Switch/1
  HDL Counter/1 -> counter/1
  a/1 -> Multiply-Add/1
  HDL Counter/2 -> Delay1/1

== system gm_Model/DUT_FixP/Deblurring/Chebyshev/LaplacianMultiply ==
  Image_in : Inport
  Delay : Delay  DelayLength=1
  LapMultiplyFi : MATLAB Function  TreatAsAtomicUnit=on
  Image_out : Outport
  wires:
  LapMultiplyFi/1(out) -> Image_out/1
  Delay/1 -> LapMultiplyFi/1(image_in)
  Image_in/1 -> Delay/1

== system gm_Model/DUT_FixP/Goertzel/DataValidDownsampler/RisingEdgeDetector ==
  In1 : Inport
  AND : Logic  IconShape=distinctive  AllPortsSameDT=off  OutDataTypeStr=boolean
  Delay1 : Delay  DelayLength=1
  NOT : Logic  Operator=NOT  IconShape=distinctive  AllPortsSameDT=off  OutDataTypeStr=boolean
  Out1 : Outport
  wires:
  Delay1/1 -> NOT/1
  AND/1 -> Out1/1
  NOT/1 -> AND/1
  In1/1 -> AND/2, Delay1/1

== system gm_Model/DUT_FixP/Goertzel/EnabledGoertzel/Goertzel filter ==
  u : Inport
  Reset : Inport  Port=2
  For All Bins Filter : Subsystem  TreatAsAtomicUnit=on  mask{cos_omega=cos_omega_fixp, exp_omega=exp_omega_fixp}
  State Control : StateControl  StateControl=Synchronous
  Sum of Elements : Sum  Inputs=+  CollapseMode=Specified dimension  OutDataTypeStr=Inherit: Same as accumulator
  Out1 : Outport  VectorParamsAs1DForOutWhenUnconnected=off
  wires:
  Reset/1 -> For All Bins Filter/2(Reset)
  For All Bins Filter/1(Out1) -> Sum of Elements/1
  Sum of Elements/1 -> Out1/1
  u/1 -> For All Bins Filter/1(In)

== system gm_Model/DUT_FixP/Goertzel/EnabledGoertzel/Symmetric Hann ==
  u : Inport
  Compare To Constant : simulink/Logic and Bit Operations/Compare To Constant  relop=<  const=nf/2  OutDataTypeStr=boolean
  Constant : Constant  Value=nf-1  OutDataTypeStr=Inherit: Inherit via back propagation  SampleTime=-1
  Hann : Lookup_n-D  NumberOfTableDimensions=1  LookupTableObject=''  BreakpointsSpecification=Even spacing  BreakpointsForDimension1=[1:200]  BreakpointsForDimension1FirstPoint=0  BreakpointsForDimension2FirstPoint=10  BreakpointsForDimension2Spacing=12  IndexSearchMethod=Evenly spaced points  Table=hann_table_fixp  TableDataTypeStr=Inherit: Inherit from 'Table data'  InterpMethod=Flat  DiagnosticForOutOfRangeInput=Error  InternalRulePriority=Speed  OutDataTypeStr=fixdt(0,fixp_input_ws,fixp_input_ws)  RndMeth=Simplest
  Sum : Sum  Inputs=|-+  OutDataTypeStr=Inherit: Same as accumulator
  Switch : Switch  Criteria=u2 ~= 0  SaturateOnIntegerOverflow=off  InputSameDT=off
  Out1 : Outport
  wires:
  Hann/1 -> Out1/1
  Compare To Constant/1 -> Switch/2
  Switch/1 -> Hann/1
  Constant/1 -> Sum/2
  Sum/1 -> Switch/3
  u/1 -> Sum/1, Compare To Constant/1, Switch/1

== system gm_Model/DUT_Test/CrossCor/streaming_partition_streamed/Serializer_Subnetwork ==
  in0 : Inport  OutDataTypeStr=fixdt(1, 18, 13)  PortDimensions=[2304 1]  SampleTime=3.125e-07
      settings: SignalType=complex
  in1 : Inport  Port=2  OutDataTypeStr=fixdt(0, 6, 0)  SampleTime=3.125e-07
  ratechange_splitcomp : Demux  Outputs=48
  splitcomp_multiport : MultiPortSwitch  DataPortOrder=Zero-based contiguous  Inputs=48  DiagnosticForDefault=None  zeroidx=on  OutDataTypeStr=fixdt(1, 18, 13)  SampleTime=3.125e-07  SaturateOnIntegerOverflow=off  InputSameDT=off
  out0 : Outport  OutDataTypeStr=fixdt(1, 18, 13)  PortDimensions=[48]  SampleTime=3.125e-07
      settings: SignalType=complex
  wires:
  in1/1 -> splitcomp_multiport/1
  ratechange_splitcomp/46 -> splitcomp_multiport/47
  ratechange_splitcomp/45 -> splitcomp_multiport/46
  ratechange_splitcomp/18 -> splitcomp_multiport/19
  in0/1 -> ratechange_splitcomp/1
  ratechange_splitcomp/1 -> splitcomp_multiport/2
  ratechange_splitcomp/2 -> splitcomp_multiport/3
  ratechange_splitcomp/5 -> splitcomp_multiport/6
  ratechange_splitcomp/3 -> splitcomp_multiport/4
  ratechange_splitcomp/4 -> splitcomp_multiport/5
  ratechange_splitcomp/43 -> splitcomp_multiport/44
  ratechange_splitcomp/6 -> splitcomp_multiport/7
  ratechange_splitcomp/26 -> splitcomp_multiport/27
  ratechange_splitcomp/7 -> splitcomp_multiport/8
  ratechange_splitcomp/15 -> splitcomp_multiport/16
  ratechange_splitcomp/8 -> splitcomp_multiport/9
  ratechange_splitcomp/47 -> splitcomp_multiport/48
  ratechange_splitcomp/25 -> splitcomp_multiport/26
  ratechange_splitcomp/24 -> splitcomp_multiport/25
  ratechange_splitcomp/23 -> splitcomp_multiport/24
  ratechange_splitcomp/9 -> splitcomp_multiport/10
  ratechange_splitcomp/10 -> splitcomp_multiport/11
  ratechange_splitcomp/35 -> splitcomp_multiport/36
  ratechange_splitcomp/22 -> splitcomp_multiport/23
  ratechange_splitcomp/11 -> splitcomp_multiport/12
  ratechange_splitcomp/21 -> splitcomp_multiport/22
  ratechange_splitcomp/12 -> splitcomp_multiport/13
  ratechange_splitcomp/13 -> splitcomp_multiport/14
  ratechange_splitcomp/14 -> splitcomp_multiport/15
  ratechange_splitcomp/16 -> splitcomp_multiport/17
  ratechange_splitcomp/40 -> splitcomp_multiport/41
  ratechange_splitcomp/39 -> splitcomp_multiport/40
  ratechange_splitcomp/17 -> splitcomp_multiport/18
  ratechange_splitcomp/20 -> splitcomp_multiport/21
  ratechange_splitcomp/19 -> splitcomp_multiport/20
  ratechange_splitcomp/28 -> splitcomp_multiport/29
  ratechange_splitcomp/27 -> splitcomp_multiport/28
  ratechange_splitcomp/29 -> splitcomp_multiport/30
  ratechange_splitcomp/30 -> splitcomp_multiport/31
  ratechange_splitcomp/34 -> splitcomp_multiport/35
  ratechange_splitcomp/32 -> splitcomp_multiport/33
  ratechange_splitcomp/31 -> splitcomp_multiport/32
  ratechange_splitcomp/33 -> splitcomp_multiport/34
  ratechange_splitcomp/36 -> splitcomp_multiport/37
  ratechange_splitcomp/37 -> splitcomp_multiport/38
  ratechange_splitcomp/38 -> splitcomp_multiport/39
  ratechange_splitcomp/44 -> splitcomp_multiport/45
  ratechange_splitcomp/41 -> splitcomp_multiport/42
  ratechange_splitcomp/42 -> splitcomp_multiport/43
  ratechange_splitcomp/48 -> splitcomp_multiport/49
  splitcomp_multiport/1 -> out0/1

== system gm_Model/DUT_Test/CrossCor/streaming_partition_streamed/c3_Product_out1_bypass ==
  in0 : Inport  OutDataTypeStr=fixdt(1, 18, 13)  PortDimensions=[48]  SampleTime=3.125e-07
      settings: SignalType=complex
  in1 : Inport  Port=2  OutDataTypeStr=boolean  SampleTime=3.125e-07
  c3_Product_out1_enb : Switch  Criteria=u2 ~= 0  Threshold=double(0)  OutDataTypeStr=fixdt(1, 18, 13)  SampleTime=3.125e-07  SaturateOnIntegerOverflow=off  InputSameDT=off
  c3_Product_out1_state : Delay  DelayLength=double(1)  InitialCondition=0  SampleTime=3.125e-07
  out0 : Outport  OutDataTypeStr=fixdt(1, 18, 13)  PortDimensions=[48]  SampleTime=3.125e-07
      settings: SignalType=complex
  wires:
  in1/1 -> c3_Product_out1_enb/2
  in0/1 -> c3_Product_out1_enb/1
  c3_Product_out1_state/1 -> c3_Product_out1_enb/3
  c3_Product_out1_enb/1 -> c3_Product_out1_state/1, out0/1

== system gm_Model/DUT_Test/CrossCor/streaming_partition_streamed/counter ==
  globalSchedule : EnablePort  OutDataTypeStr=boolean
  ctr_0_47 : hdlsllib/Sources/HDL Counter  CountType=Count limited  CountInit=double(0)  CountStep=double(1)  CountMax=double(47)  CountFromType=Initial value  CountFrom=double(0)  CountResetPort=off  CountLoadPort=off  CountEnbPort=off  CountDirPort=off  CountHitOutputPort=off  CountDataType=Unsigned  CountWordLen=6  CountFracLen=0  CountSampTime=3.125e-07
  out0 : Outport  OutDataTypeStr=fixdt(0, 6, 0)  SampleTime=3.125e-07  InitialOutput=0
  wires:
  ctr_0_47/1 -> out0/1

== system gm_Model/DUT_Test/CrossCor/streaming_partition_streamed/tappedDelay ==
  in0 : Inport  OutDataTypeStr=fixdt(1, 18, 13)  PortDimensions=[48]  SampleTime=3.125e-07
      settings: SignalType=complex
  globalSchedule : EnablePort  OutDataTypeStr=boolean
  StateControl : StateControl  StateControl=Synchronous
  tapped_delay : hdlstreaminglib/TappedDelay_VectorInputs  NumDelays=double(47)  vinit=0  DelayOrder=Oldest  includeCurrent=off
  out0 : Outport  OutDataTypeStr=fixdt(1, 18, 13)  PortDimensions=[2256]  SampleTime=3.125e-07  InitialOutput=0
      settings: SignalType=complex
  wires:
  in0/1 -> tapped_delay/1
  tapped_delay/1 -> out0/1
